simulink model "ex2"  (R2015a)
settings: Solver=ode45  StartTime=0.0  StopTime=10.0  RelTol=1e-3
settings Model: Creator=ayush  LastModifiedBy=ayush

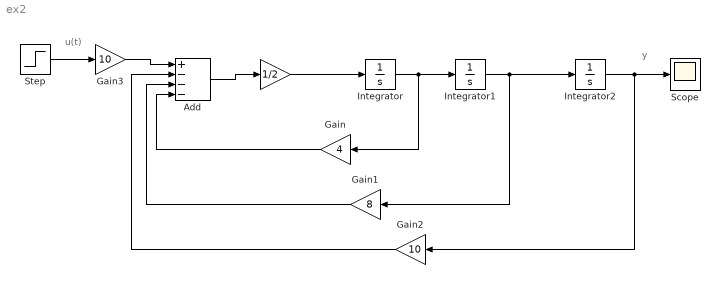
== system ex2 ==
  note: u(t)
  note: y
  " " : Gain  Gain=1/2
  Add : Sum  Inputs=+---
  Gain : Gain  Gain=4
  Gain1 : Gain  Gain=8
  Gain2 : Gain  Gain=10
  Gain3 : Gain  Gain=10
  Integrator : Integrator
  Integrator1 : Integrator
  Integrator2 : Integrator
  Scope : Scope
  Step : Step  Time=0  After=10  SampleTime=0
  wires:
  Add/1 -> " "/1
  " "/1 -> Integrator/1
  Integrator/1 -> Gain/1, Integrator1/1
  Integrator1/1 -> Integrator2/1, Gain1/1
  Gain/1 -> Add/4
  Gain1/1 -> Add/3
  Step/1 -> Gain3/1
  Integrator2/1 -> Gain2/1, Scope/1
  Gain2/1 -> Add/2
  Gain3/1 -> Add/1
